simulink model "Sursa_stabilizata_rugulator"  (R2020a)
settings: Solver=VariableStepAuto  StartTime=0.0  StopTime=0.01  RelTol=1e-3
settings Model: Creator=Stefi  LastModifiedBy=Stefi

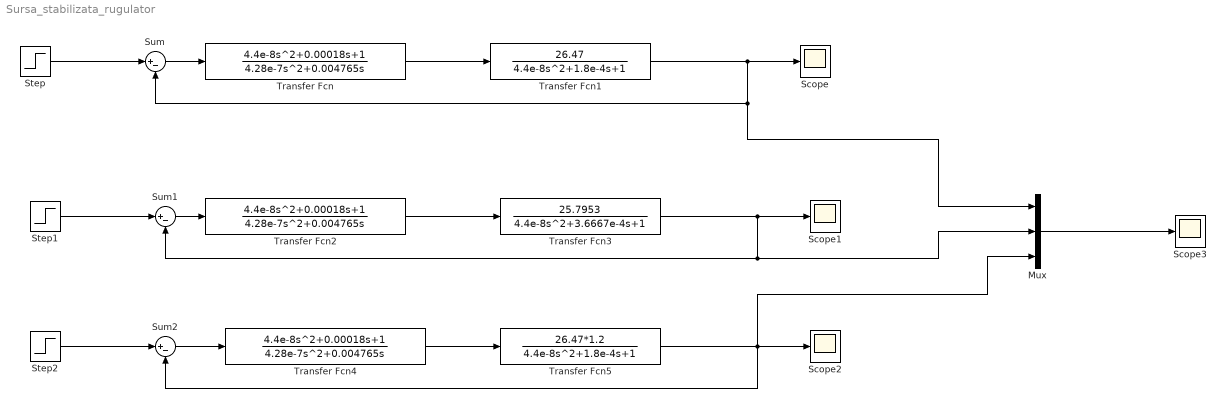
== system Sursa_stabilizata_rugulator ==
  Mux : Mux  Inputs=3
  Scope{,1..3} (4 alike) : Scope
  Step : Step  Time=0  After=2.65  SampleTime=0
  Step1 : Step  Time=0  After=2.65  SampleTime=0
  Step2 : Step  Time=0  After=2.65  SampleTime=0
  Sum : Sum  Inputs=|+-
  Sum1 : Sum  Inputs=|+-
  Sum2 : Sum  Inputs=|+-
  Transfer Fcn : TransferFcn  Numerator=[4.4e-8 0.00018 1]  Denominator=[4.28e-7 0.004765 0]
  Transfer Fcn1 : TransferFcn  Numerator=26.47  Denominator=[4.4e-8 1.8e-4 1]
  Transfer Fcn2 : TransferFcn  Numerator=[4.4e-8 0.00018 1]  Denominator=[4.28e-7 0.004765 0]
  Transfer Fcn3 : TransferFcn  Numerator=25.7953  Denominator=[4.4e-8 3.6667e-4 1]
  Transfer Fcn4 : TransferFcn  Numerator=[4.4e-8 0.00018 1]  Denominator=[4.28e-7 0.004765 0]
  Transfer Fcn5 : TransferFcn  Numerator=26.47*1.2  Denominator=[4.4e-8 1.8e-4 1]
  wires:
  Transfer Fcn1/1 -> Scope/1, Mux/1, Sum/2
  Sum/1 -> Transfer Fcn/1
  Transfer Fcn/1 -> Transfer Fcn1/1
  Step/1 -> Sum/1
  Step1/1 -> Sum1/1
  Transfer Fcn3/1 -> Scope1/1, Mux/2, Sum1/2
  Step2/1 -> Sum2/1
  Transfer Fcn4/1 -> Transfer Fcn5/1
  Mux/1 -> Scope3/1
  Transfer Fcn2/1 -> Transfer Fcn3/1
  Sum1/1 -> Transfer Fcn2/1
  Sum2/1 -> Transfer Fcn4/1
  Transfer Fcn5/1 -> Mux/3, Sum2/2, Scope2/1
